simulink model "Inverted_Wedge_2016a"  (R2017b)
settings: Solver=ode4  StartTime=0.0  StopTime=40  FixedStep=0.01  RelTol=1e-3
libraries: fuzblock x1
settings Model: Creator=Do Hoang Thai Duong  LastModifiedBy=phamt
settings DataIOCC: ReturnWorkspaceOutputs=on
settings OptimizationCC: LifeSpan=inf
settings DebuggingCC: SFExecutionAtInitializationDiag=none
settings SFSimCC: SimUseLocalCustomCode=on
settings RTWCC: RTWUseLocalCustomCode=on
settings CodeAppCC: StateflowObjectComments=on

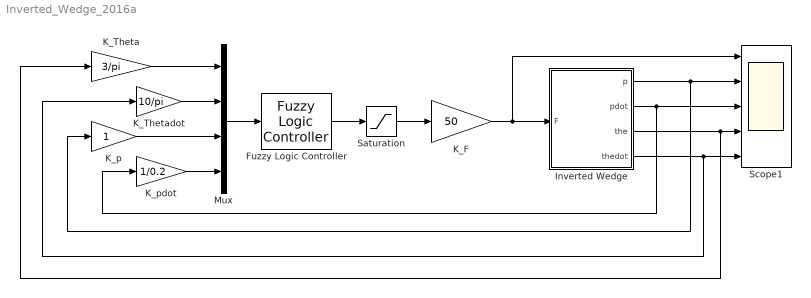
== system Inverted_Wedge_2016a ==
  Fuzzy Logic Controller : fuzblock/Fuzzy Logic  Controller  FIS='bai_FIS.fis'  OutputSampleNumber=101  DataType=double  FuzzifiedInputs=off  RuleFiringStrengths=off  RuleOutputs=off  AggregatedOutputs=off  SimulateUsing=Interpreted execution
  Inverted Wedge : Subsystem  mask{mw=3.8, mc=0.53, J=0.14, h=0.065, c=0.027, b1=0.048, b2=0.045, g=9.81, p0=0.01, pdot0=0, the0=pi/18, thedot0=0}
  K_F : Gain  Gain=50
  K_Theta : Gain  Gain=3/pi
  K_Thetadot : Gain  Gain=10/pi
  K_p : Gain
  K_pdot : Gain  Gain=1/0.2
  Mux : Mux
  Saturation : Saturate  UpperLimit=1  LowerLimit=-1
  Scope1 : Scope  NumInputPorts=5
  wires:
  Saturation/1 -> K_F/1
  Fuzzy Logic Controller/1 -> Saturation/1
  K_F/1 -> Scope1/1, Inverted Wedge/1(F)
  Mux/1 -> Fuzzy Logic Controller/1
  K_pdot/1 -> Mux/4
  K_p/1 -> Mux/3
  K_Thetadot/1 -> Mux/2
  K_Theta/1 -> Mux/1
  Inverted Wedge/3(the) -> K_Theta/1, Scope1/4
  Inverted Wedge/4(thedot) -> K_Thetadot/1, Scope1/5
  Inverted Wedge/1(p) -> K_p/1, Scope1/2
  Inverted Wedge/2(pdot) -> K_pdot/1, Scope1/3

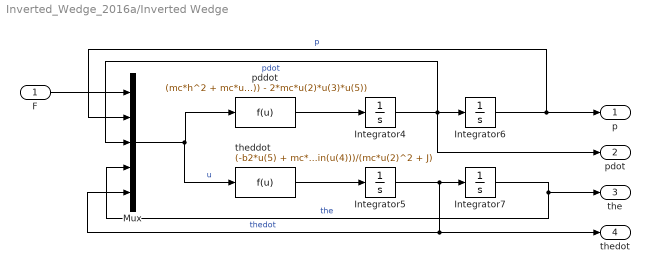
== system Inverted_Wedge_2016a/Inverted Wedge ==
  F : Inport
  Integrator4 : Integrator  InitialCondition=pdot0
  Integrator5 : Integrator  InitialCondition=thedot0
  Integrator6 : Integrator  InitialCondition=p0
  Integrator7 : Integrator  InitialCondition=the0
  Mux : Mux  Inputs=5
  pddot : Fcn  Expr=(mc*h^2 + mc*u(2)^2 + J)*(u(1) - b1*u(3) + mc*u(2)*u(5)^2 + mc*g*sin(u(4)))/(mc^2*u(2)^2 + mc*J) - ((mc*h)/(mc^2*u(2)^2 + mc*J))*(-b2*u(5) + mc*g*h*sin(u(4)) + mc*g*u(2)*cos(u(4)) + mw*g*c*sin(u(4)) - 2*mc*u(2)*u(3)*u(5))
  theddot : Fcn  Expr=(-b2*u(5) + mc*g*h*sin(u(4)) + mc*g*u(2)*cos(u(4)) + mw*g*c*sin(u(4)) - 2*mc*u(2)*u(3)*u(5))/(mc*u(2)^2 + J) - h*(u(1) - b1*u(3) + mc*u(2)*u(5)^2 + mc*g*sin(u(4)))/(mc*u(2)^2 + J)
  p : Outport
  pdot : Outport  Port=2
  the : Outport  Port=3
  thedot : Outport  Port=4
  wires:
  Integrator5/1 -> Mux/5, thedot/1, Integrator7/1  "thedot"
  pddot/1 -> Integrator4/1
  theddot/1 -> Integrator5/1
  F/1 -> Mux/1
  Mux/1 -> theddot/1, pddot/1  "u"
  Integrator4/1 -> Mux/3, pdot/1, Integrator6/1  "pdot"
  Integrator6/1 -> Mux/2, p/1  "p"
  Integrator7/1 -> Mux/4, the/1  "the"
